simulink library "MEKF_Inputs_lib"  (R2018b)
settings: Solver=VariableStepAuto  StartTime=0.0  StopTime=10.0  RelTol=1e-3
undefined symbols (not defined in the file or in its folder): simParams, sunsensor_2body_lib, sunsensor_body_rad
libraries: aerolibutil x1
settings Model: Creator=kylle  LastModifiedBy=kylle

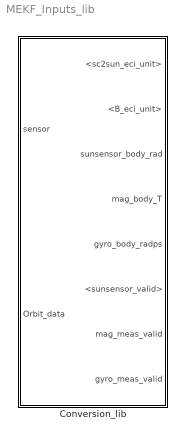
== system MEKF_Inputs_lib ==
  Conversion_lib : Subsystem

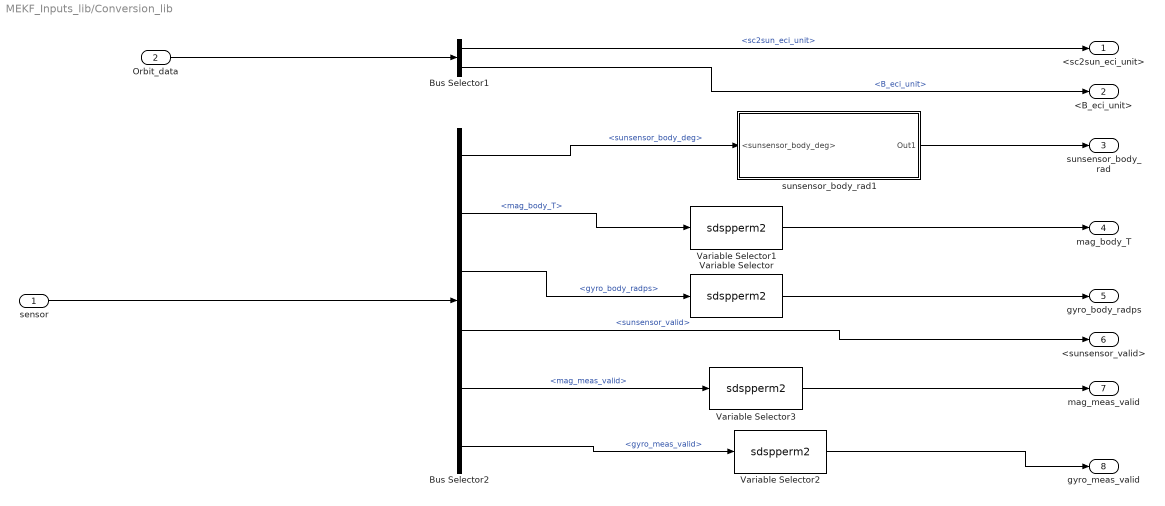
== system MEKF_Inputs_lib/Conversion_lib ==
  sensor : Inport
  Orbit_data : Inport  Port=2
  Bus Selector1 : BusSelector  OutputSignals=sc2sun_eci_unit,B_eci_unit
  Bus Selector2 : BusSelector  OutputSignals=sunsensor_body_deg,mag_body_T,gyro_body_radps,sunsensor_valid,mag_meas_valid,gyro_meas_valid
  Variable Selector : S-Function  AncestorBlock=dspindex/Variable Selector  FunctionName=sdspperm2  Parameters=1,NumInputs, rowsOrCols, IdxMode, Elements, FillMode, FillValues, errmode, 0, ZerOneIdxMode  SFunctionDeploymentMode=off  EnableBusSupport=off  mask(Variable Selector){NumInputs=1, rowsOrCols=Columns, IdxMode=Fixed, Elements=[1], ZerOneIdxMode=One-based, errmode=Clip Index, FillMode=off, FillValues=0, ShowPortLabels=off}
      mask prompts: NumInputs "Number of input signals:"; rowsOrCols "Select:"; IdxMode "Selector mode:"; ZerOneIdxMode "Index mode:"; errmode "Invalid index:"; FillMode "Fill empty spaces in outputs (for logical indexing)"; FillValues "Fill values:"; ShowPortLabels "Unused:"
      mask help:
      | Selects and/or reorders the rows or columns of the input according to a specified vector of indices (the indices need not be unique). The 'Selector mode' parameter determines whether the block uses the same indices for every input ('Fixed'), or uses different indices for every input ('Variable'). When set to 'Variable', you provide the vector of indices through an input port.
      |
      | When the indices are of Boolean data type the block performs logical indexing.
      mask init:
      | if ~isempty(NumInputs) && isfinite(NumInputs) && ~isnan(NumInputs) ...
      |  && isscalar(NumInputs) && isreal(NumInputs) && (NumInputs>0)
      |     maskdisplay = ['disp([''Select\n' get_param(gcbh, 'rowsOrCols') ''']);'];
      | 
      |     for i=1:NumInputs
      |         istr = int2str(i);
      |         maskdisplay = [maskdisplay 'port_label(''input'',' istr, ',''In' istr ''');'];
      |         maskdisplay = [maskdisplay 'port_label(''output'',' istr, ',''Out' istr ''');'];
      |     end
      | 
      |     if  IdxMode==2
      |         istr = int2str(NumInputs+1);
      |         maskdisplay = [maskdisplay 'port_label(''input'',' istr, ',''Idx'');'];
      |     end
      |     set_param(gcb, 'MaskDisplay', maskdisplay);
      | end
      mask Help: eval('blocksethelp');
      mask TypeOptions rowsOrCols: Rows | Columns
      mask TypeOptions IdxMode: Fixed | Variable
      mask Callback IdxMode: dspblkperm2;
      mask TypeOptions ZerOneIdxMode: Zero-based | One-based
      mask TypeOptions errmode: Clip Index | Clip and Warn | Generate Error
      mask Callback FillMode: dspblkperm2;
      mask Display: disp(['Select\nColumns']);port_label('input',1,'In1');port_label('output',1,'Out1');
  Variable Selector1 : S-Function  AncestorBlock=dspindex/Variable Selector  FunctionName=sdspperm2  Parameters=1,NumInputs, rowsOrCols, IdxMode, Elements, FillMode, FillValues, errmode, 0, ZerOneIdxMode  SFunctionDeploymentMode=off  EnableBusSupport=off  mask(Variable Selector){NumInputs=1, rowsOrCols=Columns, IdxMode=Fixed, Elements=[1], ZerOneIdxMode=One-based, errmode=Clip Index, FillMode=off, FillValues=0, ShowPortLabels=off}
      mask prompts: NumInputs "Number of input signals:"; rowsOrCols "Select:"; IdxMode "Selector mode:"; ZerOneIdxMode "Index mode:"; errmode "Invalid index:"; FillMode "Fill empty spaces in outputs (for logical indexing)"; FillValues "Fill values:"; ShowPortLabels "Unused:"
      mask help:
      | Selects and/or reorders the rows or columns of the input according to a specified vector of indices (the indices need not be unique). The 'Selector mode' parameter determines whether the block uses the same indices for every input ('Fixed'), or uses different indices for every input ('Variable'). When set to 'Variable', you provide the vector of indices through an input port.
      |
      | When the indices are of Boolean data type the block performs logical indexing.
      mask init: same as MEKF_Inputs_lib/Conversion_lib/Variable Selector
      mask Help: eval('blocksethelp');
      mask TypeOptions rowsOrCols: Rows | Columns
      mask TypeOptions IdxMode: Fixed | Variable
      mask Callback IdxMode: dspblkperm2;
      mask TypeOptions ZerOneIdxMode: Zero-based | One-based
      mask TypeOptions errmode: Clip Index | Clip and Warn | Generate Error
      mask Callback FillMode: dspblkperm2;
      mask Display: disp(['Select\nColumns']);port_label('input',1,'In1');port_label('output',1,'Out1');
  Variable Selector2 : S-Function  AncestorBlock=dspindex/Variable Selector  FunctionName=sdspperm2  Parameters=1,NumInputs, rowsOrCols, IdxMode, Elements, FillMode, FillValues, errmode, 0, ZerOneIdxMode  SFunctionDeploymentMode=off  EnableBusSupport=off  mask(Variable Selector){NumInputs=1, rowsOrCols=Rows, IdxMode=Fixed, Elements=[1], ZerOneIdxMode=One-based, errmode=Clip Index, FillMode=off, FillValues=0, ShowPortLabels=off}
      mask prompts: NumInputs "Number of input signals:"; rowsOrCols "Select:"; IdxMode "Selector mode:"; ZerOneIdxMode "Index mode:"; errmode "Invalid index:"; FillMode "Fill empty spaces in outputs (for logical indexing)"; FillValues "Fill values:"; ShowPortLabels "Unused:"
      mask help:
      | Selects and/or reorders the rows or columns of the input according to a specified vector of indices (the indices need not be unique). The 'Selector mode' parameter determines whether the block uses the same indices for every input ('Fixed'), or uses different indices for every input ('Variable'). When set to 'Variable', you provide the vector of indices through an input port.
      |
      | When the indices are of Boolean data type the block performs logical indexing.
      mask init: same as MEKF_Inputs_lib/Conversion_lib/Variable Selector
      mask Help: eval('blocksethelp');
      mask TypeOptions rowsOrCols: Rows | Columns
      mask TypeOptions IdxMode: Fixed | Variable
      mask Callback IdxMode: dspblkperm2;
      mask TypeOptions ZerOneIdxMode: Zero-based | One-based
      mask TypeOptions errmode: Clip Index | Clip and Warn | Generate Error
      mask Callback FillMode: dspblkperm2;
      mask Display: disp(['Select\nRows']);port_label('input',1,'In1');port_label('output',1,'Out1');
  Variable Selector3 : S-Function  AncestorBlock=dspindex/Variable Selector  FunctionName=sdspperm2  Parameters=1,NumInputs, rowsOrCols, IdxMode, Elements, FillMode, FillValues, errmode, 0, ZerOneIdxMode  SFunctionDeploymentMode=off  EnableBusSupport=off  mask(Variable Selector){NumInputs=1, rowsOrCols=Rows, IdxMode=Fixed, Elements=[1], ZerOneIdxMode=One-based, errmode=Clip Index, FillMode=off, FillValues=0, ShowPortLabels=off}
      mask prompts: NumInputs "Number of input signals:"; rowsOrCols "Select:"; IdxMode "Selector mode:"; ZerOneIdxMode "Index mode:"; errmode "Invalid index:"; FillMode "Fill empty spaces in outputs (for logical indexing)"; FillValues "Fill values:"; ShowPortLabels "Unused:"
      mask help:
      | Selects and/or reorders the rows or columns of the input according to a specified vector of indices (the indices need not be unique). The 'Selector mode' parameter determines whether the block uses the same indices for every input ('Fixed'), or uses different indices for every input ('Variable'). When set to 'Variable', you provide the vector of indices through an input port.
      |
      | When the indices are of Boolean data type the block performs logical indexing.
      mask init: same as MEKF_Inputs_lib/Conversion_lib/Variable Selector
      mask Help: eval('blocksethelp');
      mask TypeOptions rowsOrCols: Rows | Columns
      mask TypeOptions IdxMode: Fixed | Variable
      mask Callback IdxMode: dspblkperm2;
      mask TypeOptions ZerOneIdxMode: Zero-based | One-based
      mask TypeOptions errmode: Clip Index | Clip and Warn | Generate Error
      mask Callback FillMode: dspblkperm2;
      mask Display: disp(['Select\nRows']);port_label('input',1,'In1');port_label('output',1,'Out1');
  sunsensor_body_rad1 : Subsystem  AncestorBlock=sunsensor_2body_lib/sunsensor_body_rad
  <sc2sun_eci_unit> : Outport
  <B_eci_unit> : Outport  Port=2
  sunsensor_body_rad : Outport  Port=3
  mag_body_T : Outport  Port=4
  gyro_body_radps : Outport  Port=5
  <sunsensor_valid> : Outport  Port=6
  mag_meas_valid : Outport  Port=7
  gyro_meas_valid : Outport  Port=8
  wires:
  Bus Selector2/3 -> Variable Selector/1  "<gyro_body_radps>"
  Bus Selector1/2 -> <B_eci_unit>/1  "<B_eci_unit>"
  Bus Selector2/1 -> sunsensor_body_rad1/1(<sunsensor_body_deg>)  "<sunsensor_body_deg>"
  Bus Selector2/2 -> Variable Selector1/1  "<mag_body_T>"
  sunsensor_body_rad1/1(Out1) -> sunsensor_body_rad/1
  Bus Selector2/5 -> Variable Selector3/1  "<mag_meas_valid>"
  Bus Selector2/6 -> Variable Selector2/1  "<gyro_meas_valid>"
  sensor/1 -> Bus Selector2/1
  Variable Selector1/1 -> mag_body_T/1
  Variable Selector2/1 -> gyro_meas_valid/1
  Bus Selector1/1 -> <sc2sun_eci_unit>/1  "<sc2sun_eci_unit>"
  Bus Selector2/4 -> <sunsensor_valid>/1  "<sunsensor_valid>"
  Orbit_data/1 -> Bus Selector1/1
  Variable Selector/1 -> gyro_body_radps/1
  Variable Selector3/1 -> mag_meas_valid/1

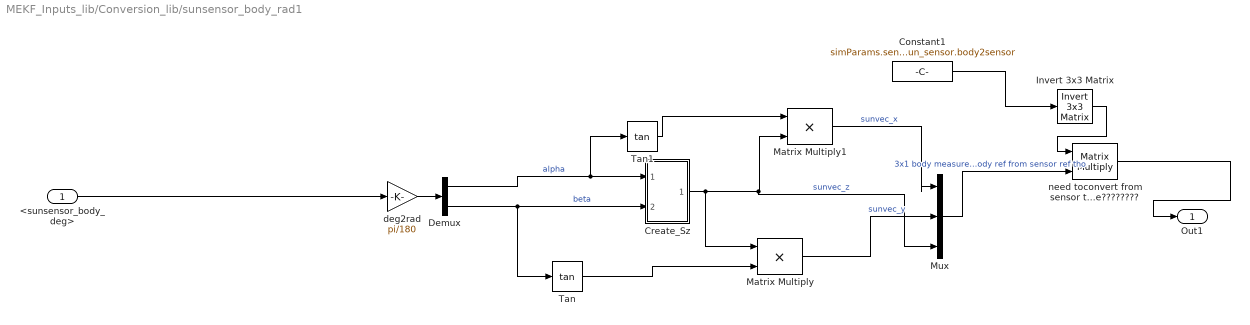
== system MEKF_Inputs_lib/Conversion_lib/sunsensor_body_rad1 ==
  <sunsensor_body_deg> : Inport
  Constant1 : Constant  Value=simParams.sensors.sun_sensor.body2sensor
  Create_Sz : Subsystem
  Demux : Demux  Outputs=2
  Invert 3x3 Matrix : aerolibutil/Invert  3x3 Matrix
  Matrix Multiply : Product
  Matrix Multiply1 : Product
  Mux : Mux  Inputs=3
  Tan : Trigonometry  Operator=tan
  Tan1 : Trigonometry  Operator=tan
  deg2rad : Gain  Gain=pi/180
  need toconvert from sensor to body frame???????? : Product  Multiplication=Matrix(*)
  Out1 : Outport
  wires:
  Tan/1 -> Matrix Multiply/2
  Demux/1 -> Tan1/1, Create_Sz/1(alpha)  "alpha"
  Matrix Multiply/1 -> Mux/2  "sunvec_y"
  Create_Sz/1(Out1) -> Mux/3, Matrix Multiply1/2, Matrix Multiply/1  "sunvec_z"
  Demux/2 -> Tan/1, Create_Sz/2(beta)  "beta"
  Tan1/1 -> Matrix Multiply1/1
  deg2rad/1 -> Demux/1
  Matrix Multiply1/1 -> Mux/1  "sunvec_x"
  <sunsensor_body_deg>/1 -> deg2rad/1
  Constant1/1 -> Invert 3x3 Matrix/1
  Invert 3x3 Matrix/1 -> need toconvert from sensor to body frame????????/1
  Mux/1 -> need toconvert from sensor to body frame????????/2  "3x1 body measurements from sun sensor (possibly need to change into body ref from sensor ref tho"
  need toconvert from sensor to body frame????????/1 -> Out1/1

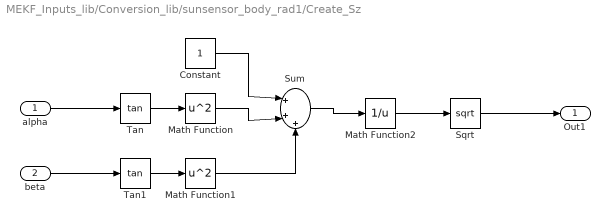
== system MEKF_Inputs_lib/Conversion_lib/sunsensor_body_rad1/Create_Sz ==
  alpha : Inport
  beta : Inport  Port=2
  Constant : Constant
  Math Function : Math  Operator=square  SaturateOnIntegerOverflow=on
  Math Function1 : Math  Operator=square  SaturateOnIntegerOverflow=on
  Math Function2 : Math  Operator=reciprocal  SaturateOnIntegerOverflow=on
  Sqrt : Sqrt  SaturateOnIntegerOverflow=on
  Sum : Sum  Inputs=|+++
  Tan : Trigonometry  Operator=tan
  Tan1 : Trigonometry  Operator=tan
  Out1 : Outport
  wires:
  Constant/1 -> Sum/1
  Sum/1 -> Math Function2/1
  Tan/1 -> Math Function/1
  Math Function/1 -> Sum/2
  Math Function2/1 -> Sqrt/1
  Tan1/1 -> Math Function1/1
  alpha/1 -> Tan/1
  beta/1 -> Tan1/1
  Math Function1/1 -> Sum/3
  Sqrt/1 -> Out1/1
